simulink model "ATRIAS_vnmc"  (R2015a)
settings: Solver=ode45  StartTime=0.0  StopTime=60  FixedStep=1e-3  MinStep=1e-6  RelTol=1e-3  AbsTol=1e-4
values from neighbouring files (symbols this model uses):
  initial_boom_yaw = initial_boom_yaw + delta_yaw0    [run_model.m]
  max_floor_diff = cost_fun_opts.max_floor_diff    [opt_cmaes.m]    (also in run_model.m; set_all_params_simple.m = 0)
  noise_on_off = cost_fun_opts.noise_on_off    [opt_cmaes.m]    (also in run_model.m; set_all_params_simple.m = 0)
  noise_seed = cost_fun_opts.noise_seed    [opt_cmaes.m]    (also in run_model.m; set_all_params_simple.m = 1)
  noise_variance = cost_fun_opts.noise_variance    [opt_cmaes.m]    (also in run_model.m; set_all_params_simple.m = 0.000174532925199)
  SEA_swing_ctrl_on_off = cost_fun_opts.SEA_swing_ctrl_on_off    [opt_cmaes.m]    (also in run_model.m; set_all_params_simple.m = 0)
  sim_t = simout.twalk    [run_model.m]
  steady_dist = cost_fun_opts.steady_dist    [opt_cmaes.m]    (also in run_model.m; set_all_params_simple.m = 10)
  ts_anim = 0.0333    [run_model.m]
undefined symbols (not defined in the file or in its folder): A1_notch_f1, A2_notch_f1, A_lpf_dtau, A_lpf_velocity, B1_lpf_dtau, B1_lpf_velocity, B1_notch_f1, B2_lpf_dtau, B2_lpf_velocity, B2_notch_f1, b_hmotor, b_leg_spring, b_rotor, base_color_d, boom_color_d, boom_mount_to_center_diagonal, breakaway_friction, c, c_jointstop, com_height_offset, contactThr, coulomb_friction, CtrlPar_theta0, D12_S, D12_T, d_com, ddx_max, ddy_max, delta_phi_max, delta_phi_max_buffer, delta_phi_max_dropoff, delta_phi_min, des_forward_velocity, DS_width, dtau_des_max, dtheta0_vmc, dx0_vmc, dy_max, eref, fblink_color_d, fcut_acceleration, floor_color_d, floor_tile_width, floor_zero_height, FmaxBFSH, FmaxGLU, FmaxHAM, FmaxHFL, FmaxRF, FmaxVAS, FPCtrlPar, friction_linear_zone, g, gain_nodes_sea_torque, gamma_stance_thr, gamma_swing_thr, hip_height, HIP_MTR_MAX_CONT_TORQUE, HIP_MTR_MAX_TORQUE, hshaft_color_d ... (+236)
libraries: sm_lib x280, nesl_utility x174, simulink x114, simulink_extras x58, fl_lib x16, mblibv1 x2, dspswit3 x2
(part 9 of 23)

== system ATRIAS_vnmc/control/Virtual Model Control/Flight PD ==
  R Back Gear [rad rad/s] : Inport
  R Front Gear [rad rad/s] : Inport  Port=2
  L Back Gear [rad rad/s] : Inport  Port=3
  L Front Gear [rad rad/s] : Inport  Port=4
  R Length des [m] : Inport  Port=5
  R Gamma des [m] : Inport  Port=6
  L Length des [m] : Inport  Port=7
  L Angle des [m] : Inport  Port=8
  theta [rad] : Inport  Port=9
  Avoid Hitting Mechanical Limits1 : MATLAB Function  TreatAsAtomicUnit=on
  Avoid Hitting Mechanical Limits2 : MATLAB Function  TreatAsAtomicUnit=on
  Back/Front Motor PD1 : Subsystem
  Back/Front Motor PD2 : Subsystem
  Constant{3,5,7..12} (8 alike) : Constant  Value=0
  Demux{1..4} (4 alike) : Demux  Outputs=2
  Mux{1..9,11} (10 alike) : Mux  Inputs=2
  Sum : Sum  Inputs=|+-
  Sum1 : Sum  Inputs=-+|
  Virtual Leg to Four Bar1 : MATLAB Function  TreatAsAtomicUnit=on
  Virtual Leg to Four Bar2 : MATLAB Function  TreatAsAtomicUnit=on
  R cmd [Nm] [back front] : Outport
  L cmd [Nm] [back front] : Outport  Port=2
  wires:
  Virtual Leg to Four Bar1/1(back) -> Avoid Hitting Mechanical Limits1/1(back_desired)
  Virtual Leg to Four Bar1/2(dback) -> Avoid Hitting Mechanical Limits1/2(dback_desired)
  Virtual Leg to Four Bar1/3(ddback) -> Avoid Hitting Mechanical Limits1/3(ddback_desired)
  Virtual Leg to Four Bar1/4(front) -> Avoid Hitting Mechanical Limits1/4(front_desired)
  Virtual Leg to Four Bar1/5(dfront) -> Avoid Hitting Mechanical Limits1/5(dfront_desired)
  Virtual Leg to Four Bar1/6(ddfront) -> Avoid Hitting Mechanical Limits1/6(ddfront_desired)
  Mux5/1 -> Back/Front Motor PD1/1(Desired Position [rad] [back front])
  Avoid Hitting Mechanical Limits1/2(front_cmd) -> Mux5/2
  Avoid Hitting Mechanical Limits1/1(back_cmd) -> Mux5/1
  Avoid Hitting Mechanical Limits1/3(dback_cmd) -> Mux6/1
  Avoid Hitting Mechanical Limits1/4(dfront_cmd) -> Mux6/2
  Avoid Hitting Mechanical Limits1/5(ddback_cmd) -> Mux7/1
  Avoid Hitting Mechanical Limits1/6(ddfront_cmd) -> Mux7/2
  Mux6/1 -> Back/Front Motor PD1/2(Desired Velocity [rad/s] [back front])
  Mux7/1 -> Back/Front Motor PD1/3(Desired Acceleration [rad/s^2] [back front])
  R Length des [m]/1 -> Virtual Leg to Four Bar1/1(l_leg)
  Constant7/1 -> Virtual Leg to Four Bar1/2(dl_leg)
  Constant9/1 -> Virtual Leg to Four Bar1/5(dphi)
  Constant10/1 -> Virtual Leg to Four Bar1/6(ddphi)
  Constant8/1 -> Virtual Leg to Four Bar1/3(ddl_leg)
  Mux11/1 -> Back/Front Motor PD1/5(Measured Velocity [rad/s] [back front])
  Demux2/2 -> Mux11/2
  Mux4/1 -> Back/Front Motor PD1/4(Measured Position [rad] [back front])
  Demux3/2 -> Mux11/1
  Demux3/1 -> Mux4/1
  Demux2/1 -> Mux4/2
  R Front Gear [rad rad/s]/1 -> Demux2/1
  R Back Gear [rad rad/s]/1 -> Demux3/1
  Virtual Leg to Four Bar2/1(back) -> Avoid Hitting Mechanical Limits2/1(back_desired)
  Virtual Leg to Four Bar2/2(dback) -> Avoid Hitting Mechanical Limits2/2(dback_desired)
  Virtual Leg to Four Bar2/3(ddback) -> Avoid Hitting Mechanical Limits2/3(ddback_desired)
  Virtual Leg to Four Bar2/4(front) -> Avoid Hitting Mechanical Limits2/4(front_desired)
  Virtual Leg to Four Bar2/5(dfront) -> Avoid Hitting Mechanical Limits2/5(dfront_desired)
  Virtual Leg to Four Bar2/6(ddfront) -> Avoid Hitting Mechanical Limits2/6(ddfront_desired)
  Mux3/1 -> Back/Front Motor PD2/1(Desired Position [rad] [back front])
  Avoid Hitting Mechanical Limits2/2(front_cmd) -> Mux3/2
  Avoid Hitting Mechanical Limits2/1(back_cmd) -> Mux3/1
  Avoid Hitting Mechanical Limits2/3(dback_cmd) -> Mux8/1
  Avoid Hitting Mechanical Limits2/4(dfront_cmd) -> Mux8/2
  Avoid Hitting Mechanical Limits2/5(ddback_cmd) -> Mux9/1
  Avoid Hitting Mechanical Limits2/6(ddfront_cmd) -> Mux9/2
  Mux8/1 -> Back/Front Motor PD2/2(Desired Velocity [rad/s] [back front])
  Mux9/1 -> Back/Front Motor PD2/3(Desired Acceleration [rad/s^2] [back front])
  Constant5/1 -> Virtual Leg to Four Bar2/2(dl_leg)
  Constant12/1 -> Virtual Leg to Four Bar2/5(dphi)
  Constant3/1 -> Virtual Leg to Four Bar2/6(ddphi)
  Constant11/1 -> Virtual Leg to Four Bar2/3(ddl_leg)
  Mux1/1 -> Back/Front Motor PD2/5(Measured Velocity [rad/s] [back front])
  Demux1/2 -> Mux1/2
  Mux2/1 -> Back/Front Motor PD2/4(Measured Position [rad] [back front])
  Demux4/2 -> Mux1/1
  Demux4/1 -> Mux2/1
  Demux1/1 -> Mux2/2
  L Front Gear [rad rad/s]/1 -> Demux1/1
  L Back Gear [rad rad/s]/1 -> Demux4/1
  Back/Front Motor PD1/1(Commanded Torque [Nm] [back front]) -> R cmd [Nm] [back front]/1
  Back/Front Motor PD2/1(Commanded Torque [Nm] [back front]) -> L cmd [Nm] [back front]/1
  R Gamma des [m]/1 -> Sum/1
  L Length des [m]/1 -> Virtual Leg to Four Bar2/1(l_leg)
  L Angle des [m]/1 -> Sum1/2
  Sum/1 -> Virtual Leg to Four Bar1/4(phi)
  theta [rad]/1 -> Sum/2, Sum1/1
  Sum1/1 -> Virtual Leg to Four Bar2/4(phi)

== system ATRIAS_vnmc/control/Virtual Model Control/Swing Leg Behavior1 ==
  note: Leg Angle
  note: Leg Length
  note: Open-Loop Swing Trajectory
  note: Convert to
      | four-bar angles
  note: Position control the
      | individual four bar segments
  Swing Back Gear [rad rad/s] : Inport
  Swing Front Gear [rad rad/s] : Inport  Port=2
  Stance Leg Angle [rad] : Inport  Port=3
  Horizontal Single Support Distance [m] : Inport  Port=4
  Swing Leg Length [m] : Inport  Port=5
  Swing Leg Angle [rad] : Inport  Port=6
  COM Forward Velocity [m/s] : Inport  Port=7
  theta [rad rad/s] : Inport  Port=8
  Swing Leg Stance (VMC) [0/1] : Inport  Port=9
  Avoid Hitting Mechanical Limits : MATLAB Function  TreatAsAtomicUnit=on
  Back/Front Motor PD : Subsystem
  Clock : Clock
  Clock1 : Clock
  Constant1 : Constant  Value=nominal_swing_time
  Constant10 : Constant  Value=nominal_swing_time
  Constant11 : Constant  Value=max_gamma_velocity
  Constant12 : Constant  Value=max_gamma_acceleration
  Constant13 : Constant  Value=max_leg_velocity
  Constant14 : Constant  Value=max_leg_acceleration
  Constant2 : Constant  Commented=on  Value=gamma_swing_thr
  Constant6 : Constant  Value=leg_length_retract
  Constant7 : Constant  Value=leg_length_max+leg_ground_penetration
  Constant8 : Constant  Value=2*pi-gamma_swing_thr
  Constant9 : Constant  Commented=on  Value=eps
  Demux1 : Demux
  Demux2 : Demux  Outputs=2
  Demux3 : Demux  Outputs=2
  Demux4 : Demux
  Demux5 : Demux  Outputs=2
  Detect Change : simulink/Logic and Bit Operations/Detect Change  vinit=1  InputProcessing=Inherited  OutDataTypeStr=boolean
  Divide : Product  Commented=on  Inputs=*/
  Enter Swing or Stance : simulink/Logic and Bit Operations/Detect Change  vinit=1  InputProcessing=Inherited  OutDataTypeStr=boolean
  Hold Values : Subsystem
  Hold Values1 : Subsystem
  Leg Angle Trajectory : MATLAB Function  TreatAsAtomicUnit=on
  Leg Length Trajectory : MATLAB Function  TreatAsAtomicUnit=on
  Logical Operator : Logic  Operator=OR  AllPortsSameDT=off  OutDataTypeStr=boolean
  Mux : Mux
  Mux{1..4,11} (5 alike) : Mux  Inputs=2
  Mux5 : Mux
  Saturation : Saturate  Commented=on  UpperLimit=max_swing_time/2  LowerLimit=min_swing_time/2
  Saturation1 : Saturate  Commented=on  UpperLimit=2  LowerLimit=0.5
  Saturation2 : Saturate  Commented=on  UpperLimit=max_swing_time  LowerLimit=min_swing_time
  Sum{1..2,4..5} (4 alike) : Sum  Inputs=|+-
  Sum3 : Sum  Commented=on  Inputs=|++
  Sum6 : Sum  Inputs=|++
  Sum7 : Sum  Inputs=|++
  Switch : Switch  Criteria=u2 ~= 0
  Switch1 : Switch  Commented=on  Criteria=u2 ~= 0
  Terminator1 : Terminator  Commented=on
  Vertical/Trailing Swing Leg : simulink/Logic and Bit Operations/Compare To Constant  relop=<  const=pi  OutDataTypeStr=boolean
  Virtual Leg to Four Bar : MATLAB Function  TreatAsAtomicUnit=on
  half : Gain  Gain=1/2
  Secondary Back/Front Motor Torque [Nm Nm] : Outport
  Desired Leg Length [m] : Outport  Port=2
  Desired Leg Length Velocity [m/s] : Outport  Port=3
  Desired Leg Length Acceleration [m/s^2] : Outport  Port=4
  Desired Global Leg Angle [m] : Outport  Port=5
  Desired Global Leg Angle Velocity [m/s] : Outport  Port=6
  Desired Global Leg Angle Acceleration [m/s^2] : Outport  Port=7
  wires:
  Detect Change/1 -> Logical Operator/1
  Sum7/1 -> Desired Global Leg Angle Velocity [m/s]/1
  Sum6/1 -> Desired Global Leg Angle [m]/1
  Constant2/1 -> Switch1/1
  Constant1/1 -> Mux5/2
  [ddphi_swing] -> Desired Global Leg Angle Acceleration [m/s^2]/1
  [dphi_swing] -> Sum7/1
  [phi_swing] -> Sum6/1
  [ddl_leg_swing] -> Desired Leg Length Acceleration [m/s^2]/1
  [dl_leg_swing] -> Desired Leg Length Velocity [m/s]/1
  [l_leg_swing] -> Desired Leg Length [m]/1
  half/1 -> Mux/2
  Constant13/1 -> Leg Length Trajectory/5(max_leg_velocity)
  Constant14/1 -> Leg Length Trajectory/6(max_leg_acceleration)
  Constant12/1 -> Leg Angle Trajectory/6(max_gamma_acceleration)
  Constant11/1 -> Leg Angle Trajectory/5(max_gamma_velocity)
  Sum5/1 -> [dphi_swing]
  Demux5/2 -> Sum5/2, Sum7/2
  Demux5/1 -> Sum4/2, Sum6/2
  theta [rad rad/s]/1 -> Demux5/1
  Sum4/1 -> [phi_swing]
  Stance Leg Angle [rad]/1 -> Terminator1/1
  Constant10/1 -> half/1  "dt_sat"
  Saturation1/1 -> Sum3/1
  Constant9/1 -> Sum3/2
  Sum3/1 -> Divide/2
  Constant8/1 -> Mux5/3  "target leg angle"
  Swing Leg Angle [rad]/1 -> Vertical/Trailing Swing Leg/1, Mux5/4
  Clock1/1 -> Sum1/1, Mux5/1
  Sum1/1 -> Leg Angle Trajectory/1(t)
  Demux1/1 -> Sum1/2
  Demux1/2 -> Leg Angle Trajectory/4(t_trajectory)  "tmax"
  Demux1/3 -> Leg Angle Trajectory/3(gamma_final)
  Demux1/4 -> Leg Angle Trajectory/2(gamma_initial)
  Mux5/1 -> Hold Values1/1(in)
  Hold Values1/1(out) -> Demux1/1
  Leg Angle Trajectory/3(ddgamma) -> [ddphi_swing]  "ddgamma"
  Leg Angle Trajectory/2(dgamma) -> Sum5/1
  Leg Angle Trajectory/1(gamma) -> Sum4/1  "gamma"
  Logical Operator/1 -> Hold Values/Trigger
  Horizontal Single Support Distance [m]/1 -> Divide/1
  COM Forward Velocity [m/s]/1 -> Saturation1/1
  Switch/1 -> Mux/3
  Vertical/Trailing Swing Leg/1 -> Detect Change/1, Switch/2
  Constant7/1 -> Switch/1
  Constant6/1 -> Switch/3
  Enter Swing or Stance/1 -> Hold Values1/Trigger, Logical Operator/2
  Swing Leg Stance (VMC) [0/1]/1 -> Enter Swing or Stance/1, Switch1/2
  Swing Leg Length [m]/1 -> Mux/4
  Clock/1 -> Sum2/1, Mux/1
  Sum2/1 -> Leg Length Trajectory/1(t)
  Demux4/1 -> Sum2/2
  Demux4/2 -> Leg Length Trajectory/4(t_trajectory)
  Demux4/3 -> Leg Length Trajectory/3(l_leg_final)
  Demux4/4 -> Leg Length Trajectory/2(l_leg_initial)
  Mux/1 -> Hold Values/1(in)
  Hold Values/1(out) -> Demux4/1
  Leg Length Trajectory/3(ddl_leg) -> [ddl_leg_swing]
  Leg Length Trajectory/2(dl_leg) -> [dl_leg_swing]
  Leg Length Trajectory/1(l_leg) -> [l_leg_swing]
  [ddphi_swing] -> Virtual Leg to Four Bar/6(ddphi)
  [dphi_swing] -> Virtual Leg to Four Bar/5(dphi)
  [phi_swing] -> Virtual Leg to Four Bar/4(phi)
  [ddl_leg_swing] -> Virtual Leg to Four Bar/3(ddl_leg)
  [dl_leg_swing] -> Virtual Leg to Four Bar/2(dl_leg)
  [l_leg_swing] -> Virtual Leg to Four Bar/1(l_leg)
  Mux3/1 -> Back/Front Motor PD/3(Desired Acceleration [rad/s^2] [back front])
  Mux2/1 -> Back/Front Motor PD/2(Desired Velocity [rad/s] [back front])
  Avoid Hitting Mechanical Limits/6(ddfront_cmd) -> Mux3/2
  Avoid Hitting Mechanical Limits/5(ddback_cmd) -> Mux3/1
  Avoid Hitting Mechanical Limits/4(dfront_cmd) -> Mux2/2
  Avoid Hitting Mechanical Limits/3(dback_cmd) -> Mux2/1
  Swing Back Gear [rad rad/s]/1 -> Demux3/1
  Swing Front Gear [rad rad/s]/1 -> Demux2/1
  Demux2/1 -> Mux4/2
  Avoid Hitting Mechanical Limits/1(back_cmd) -> Mux1/1
  Avoid Hitting Mechanical Limits/2(front_cmd) -> Mux1/2
  Demux3/1 -> Mux4/1
  Demux3/2 -> Mux11/1
  Mux1/1 -> Back/Front Motor PD/1(Desired Position [rad] [back front])
  Mux4/1 -> Back/Front Motor PD/4(Measured Position [rad] [back front])
  Demux2/2 -> Mux11/2
  Mux11/1 -> Back/Front Motor PD/5(Measured Velocity [rad/s] [back front])
  Virtual Leg to Four Bar/6(ddfront) -> Avoid Hitting Mechanical Limits/6(ddfront_desired)
  Virtual Leg to Four Bar/5(dfront) -> Avoid Hitting Mechanical Limits/5(dfront_desired)
  Virtual Leg to Four Bar/4(front) -> Avoid Hitting Mechanical Limits/4(front_desired)
  Virtual Leg to Four Bar/3(ddback) -> Avoid Hitting Mechanical Limits/3(ddback_desired)
  Virtual Leg to Four Bar/2(dback) -> Avoid Hitting Mechanical Limits/2(dback_desired)
  Virtual Leg to Four Bar/1(back) -> Avoid Hitting Mechanical Limits/1(back_desired)
  Back/Front Motor PD/1(Commanded Torque [Nm] [back front]) -> Secondary Back/Front Motor Torque [Nm Nm]/1

== system ATRIAS_vnmc/control/Virtual Model Control/Swing Leg Behavior2 ==
  note: Position control the
      | individual four bar segments
  note: Convert to
      | four-bar angles
  note: Open-Loop Swing Trajectory
  note: Leg Length
  note: Leg Angle
  Swing Back Gear [rad rad/s] : Inport
  Swing Front Gear [rad rad/s] : Inport  Port=2
  Stance Leg Angle [rad] : Inport  Port=3
  Horizontal Single Support Distance [m] : Inport  Port=4
  Swing Leg Length [m] : Inport  Port=5
  Swing Leg Angle [rad] : Inport  Port=6
  COM Forward Velocity [m/s] : Inport  Port=7
  theta [rad rad/s] : Inport  Port=8
  Swing Leg Stance (VMC) [0/1] : Inport  Port=9
  Add : Sum  Inputs=+-
  Add1 : Sum
  Add2 : Sum  Inputs=+-
  Avoid Hitting Mechanical Limits : MATLAB Function  TreatAsAtomicUnit=on
  Back/Front Motor PD : Subsystem
  Clock : Clock
  Clock1 : Clock
  Constant1 : Constant  Value=nominal_swing_time
  Constant10 : Constant  Value=nominal_swing_time
  Constant11 : Constant  Value=max_gamma_velocity
  Constant12 : Constant  Value=max_gamma_acceleration
  Constant13 : Constant  Value=max_leg_velocity
  Constant14 : Constant  Value=max_leg_acceleration
  Constant2 : Constant  Value=2*pi
  Constant3 : Constant  Value=hip_height
  Constant5 : Constant  Value=leg_ground_penetration
  Constant6 : Constant  Value=leg_clearance
  Constant9 : Constant  Commented=on  Value=eps
  Demux1 : Demux
  Demux2 : Demux  Outputs=2
  Demux3 : Demux  Outputs=2
  Demux4 : Demux
  Demux5 : Demux  Outputs=2
  Detect Change : simulink/Logic and Bit Operations/Detect Change  vinit=1  InputProcessing=Inherited  OutDataTypeStr=boolean
  Divide : Product  Commented=on  Inputs=*/
  Enter Swing or Stance : simulink/Logic and Bit Operations/Detect Change  vinit=1  InputProcessing=Inherited  OutDataTypeStr=boolean
  Hold Values : Subsystem
  Hold Values1 : Subsystem
  Leg Angle Trajectory : MATLAB Function  TreatAsAtomicUnit=on
  Leg Length Trajectory : MATLAB Function  TreatAsAtomicUnit=on
  Logical Operator : Logic  Operator=OR  AllPortsSameDT=off  OutDataTypeStr=boolean
  Mux : Mux
  Mux{1..4,11} (5 alike) : Mux  Inputs=2
  Mux5 : Mux
  Saturation : Saturate  Commented=on  UpperLimit=max_swing_time/2  LowerLimit=min_swing_time/2
  Saturation1 : Saturate  Commented=on  UpperLimit=2  LowerLimit=0.5
  Saturation2 : Saturate  Commented=on  UpperLimit=max_swing_time  LowerLimit=min_swing_time
  Sum{1..2,4..5} (4 alike) : Sum  Inputs=|+-
  Sum3 : Sum  Commented=on  Inputs=|++
  Sum6 : Sum  Inputs=|++
  Sum7 : Sum  Inputs=|++
  Switch : Switch  Criteria=u2 ~= 0
  Terminator1 : Terminator
  Terminator2 : Terminator
  Terminator3 : Terminator
  Vertical/Trailing Swing Leg : simulink/Logic and Bit Operations/Compare To Constant  relop=<  const=pi  OutDataTypeStr=boolean
  Virtual Leg to Four Bar : MATLAB Function  TreatAsAtomicUnit=on
  half : Gain  Gain=1/2
  Secondary Back/Front Motor Torque [Nm Nm] : Outport
  Desired Leg Length [m] : Outport  Port=2
  Desired Leg Length Velocity [m/s] : Outport  Port=3
  Desired Leg Length Acceleration [m/s^2] : Outport  Port=4
  Desired Global Leg Angle [m] : Outport  Port=5
  Desired Global Leg Angle Velocity [m/s] : Outport  Port=6
  Desired Global Leg Angle Acceleration [m/s^2] : Outport  Port=7
  wires:
  Add2/1 -> Mux5/3
  Constant2/1 -> Add2/1
  [gamma_max] -> Add2/2
  [leg_length_max] -> Add1/1
  Constant5/1 -> Add1/2
  Constant3/1 -> Add/1
  Add/1 -> Switch/3
  Back/Front Motor PD/1(Commanded Torque [Nm] [back front]) -> Secondary Back/Front Motor Torque [Nm Nm]/1
  Virtual Leg to Four Bar/1(back) -> Avoid Hitting Mechanical Limits/1(back_desired)
  Virtual Leg to Four Bar/2(dback) -> Avoid Hitting Mechanical Limits/2(dback_desired)
  Virtual Leg to Four Bar/3(ddback) -> Avoid Hitting Mechanical Limits/3(ddback_desired)
  Virtual Leg to Four Bar/4(front) -> Avoid Hitting Mechanical Limits/4(front_desired)
  Virtual Leg to Four Bar/5(dfront) -> Avoid Hitting Mechanical Limits/5(dfront_desired)
  Virtual Leg to Four Bar/6(ddfront) -> Avoid Hitting Mechanical Limits/6(ddfront_desired)
  Mux11/1 -> Back/Front Motor PD/5(Measured Velocity [rad/s] [back front])
  Demux2/2 -> Mux11/2
  Mux4/1 -> Back/Front Motor PD/4(Measured Position [rad] [back front])
  Mux1/1 -> Back/Front Motor PD/1(Desired Position [rad] [back front])
  Demux3/2 -> Mux11/1
  Demux3/1 -> Mux4/1
  Avoid Hitting Mechanical Limits/2(front_cmd) -> Mux1/2
  Avoid Hitting Mechanical Limits/1(back_cmd) -> Mux1/1
  Demux2/1 -> Mux4/2
  Swing Front Gear [rad rad/s]/1 -> Demux2/1
  Swing Back Gear [rad rad/s]/1 -> Demux3/1
  Avoid Hitting Mechanical Limits/3(dback_cmd) -> Mux2/1
  Avoid Hitting Mechanical Limits/4(dfront_cmd) -> Mux2/2
  Avoid Hitting Mechanical Limits/5(ddback_cmd) -> Mux3/1
  Avoid Hitting Mechanical Limits/6(ddfront_cmd) -> Mux3/2
  Mux2/1 -> Back/Front Motor PD/2(Desired Velocity [rad/s] [back front])
  Mux3/1 -> Back/Front Motor PD/3(Desired Acceleration [rad/s^2] [back front])
  [l_leg_swing] -> Virtual Leg to Four Bar/1(l_leg)
  [dl_leg_swing] -> Virtual Leg to Four Bar/2(dl_leg)
  [ddl_leg_swing] -> Virtual Leg to Four Bar/3(ddl_leg)
  [phi_swing] -> Virtual Leg to Four Bar/4(phi)
  [dphi_swing] -> Virtual Leg to Four Bar/5(dphi)
  [ddphi_swing] -> Virtual Leg to Four Bar/6(ddphi)
  Leg Length Trajectory/1(l_leg) -> [l_leg_swing]
  Leg Length Trajectory/2(dl_leg) -> [dl_leg_swing]
  Leg Length Trajectory/3(ddl_leg) -> [ddl_leg_swing]
  Hold Values/1(out) -> Demux4/1
  Mux/1 -> Hold Values/1(in)
  Demux4/4 -> Leg Length Trajectory/2(l_leg_initial)
  Demux4/3 -> Leg Length Trajectory/3(l_leg_final)
  Demux4/2 -> Leg Length Trajectory/4(t_trajectory)
  Demux4/1 -> Sum2/2
  Sum2/1 -> Leg Length Trajectory/1(t)
  Clock/1 -> Mux/1, Sum2/1
  Swing Leg Length [m]/1 -> Mux/4
  Swing Leg Stance (VMC) [0/1]/1 -> Enter Swing or Stance/1
  Enter Swing or Stance/1 -> Logical Operator/2, Hold Values1/Trigger
  Constant6/1 -> Add/2
  Add1/1 -> Switch/1
  Vertical/Trailing Swing Leg/1 -> Switch/2, Detect Change/1
  Switch/1 -> Mux/3
  COM Forward Velocity [m/s]/1 -> Terminator3/1
  Horizontal Single Support Distance [m]/1 -> Terminator2/1
  Logical Operator/1 -> Hold Values/Trigger
  Leg Angle Trajectory/1(gamma) -> Sum4/1  "gamma"
  Leg Angle Trajectory/2(dgamma) -> Sum5/1
  Leg Angle Trajectory/3(ddgamma) -> [ddphi_swing]  "ddgamma"
  Hold Values1/1(out) -> Demux1/1
  Mux5/1 -> Hold Values1/1(in)
  Demux1/4 -> Leg Angle Trajectory/2(gamma_initial)
  Demux1/3 -> Leg Angle Trajectory/3(gamma_final)
  Demux1/2 -> Leg Angle Trajectory/4(t_trajectory)  "tmax"
  Demux1/1 -> Sum1/2
  Sum1/1 -> Leg Angle Trajectory/1(t)
  Clock1/1 -> Sum1/1, Mux5/1
  Swing Leg Angle [rad]/1 -> Mux5/4, Vertical/Trailing Swing Leg/1
  Sum3/1 -> Divide/2
  Constant9/1 -> Sum3/2
  Saturation1/1 -> Sum3/1
  Constant10/1 -> half/1  "dt_sat"
  Stance Leg Angle [rad]/1 -> Terminator1/1
  Sum4/1 -> [phi_swing]
  theta [rad rad/s]/1 -> Demux5/1
  Demux5/1 -> Sum6/2, Sum4/2
  Demux5/2 -> Sum7/2, Sum5/2
  Sum5/1 -> [dphi_swing]
  Constant11/1 -> Leg Angle Trajectory/5(max_gamma_velocity)
  Constant12/1 -> Leg Angle Trajectory/6(max_gamma_acceleration)
  Constant14/1 -> Leg Length Trajectory/6(max_leg_acceleration)
  Constant13/1 -> Leg Length Trajectory/5(max_leg_velocity)
  half/1 -> Mux/2
  [l_leg_swing] -> Desired Leg Length [m]/1
  [dl_leg_swing] -> Desired Leg Length Velocity [m/s]/1
  [ddl_leg_swing] -> Desired Leg Length Acceleration [m/s^2]/1
  [phi_swing] -> Sum6/1
  [dphi_swing] -> Sum7/1
  [ddphi_swing] -> Desired Global Leg Angle Acceleration [m/s^2]/1
  Constant1/1 -> Mux5/2
  Sum6/1 -> Desired Global Leg Angle [m]/1
  Sum7/1 -> Desired Global Leg Angle Velocity [m/s]/1
  Detect Change/1 -> Logical Operator/1

== system ATRIAS_vnmc/control/Virtual Model Control/Swing Leg Behavior3 ==
  note: Leg Angle
  note: Leg Length
  note: Open-Loop Swing Trajectory
  note: Convert to
      | four-bar angles
  note: Position control the
      | individual four bar segments
  Swing Back Gear [rad rad/s] : Inport
  Swing Front Gear [rad rad/s] : Inport  Port=2
  Stance Leg Angle [rad] : Inport  Port=3
  Horizontal Single Support Distance [m] : Inport  Port=4
  Swing Leg Length [m] : Inport  Port=5
  Swing Leg Angle [rad] : Inport  Port=6
  COM Forward Velocity [m/s] : Inport  Port=7
  theta [rad rad/s] : Inport  Port=8
  Swing Leg Stance (VMC) [0/1] : Inport  Port=9
  Add : Sum  Inputs=+-
  Add1 : Sum  Inputs=+-
  Add2 : Sum  Inputs=+-
  Avoid Hitting Mechanical Limits : MATLAB Function  TreatAsAtomicUnit=on
  Back/Front Motor PD : Subsystem
  Clock : Clock
  Clock1 : Clock
  Constant1 : Constant  Value=nominal_swing_time
  Constant10 : Constant  Value=nominal_swing_time
  Constant11 : Constant  Value=max_gamma_velocity
  Constant12 : Constant  Value=max_gamma_acceleration
  Constant13 : Constant  Value=max_leg_velocity
  Constant14 : Constant  Value=max_leg_acceleration
  Constant2 : Constant  Value=2*pi
  Constant3 : Constant  Value=hip_height
  Constant5 : Constant  Value=leg_ground_penetration
  Constant6 : Constant  Value=leg_clearance
  Constant9 : Constant  Commented=on  Value=eps
  Demux1 : Demux
  Demux2 : Demux  Outputs=2
  Demux3 : Demux  Outputs=2
  Demux4 : Demux
  Demux5 : Demux  Outputs=2
  Detect Change : simulink/Logic and Bit Operations/Detect Change  vinit=1  InputProcessing=Inherited  OutDataTypeStr=boolean
  Divide : Product  Commented=on  Inputs=*/
  Enter Swing or Stance : simulink/Logic and Bit Operations/Detect Change  vinit=1  InputProcessing=Inherited  OutDataTypeStr=boolean
  Hold Values : Subsystem
  Hold Values1 : Subsystem
  Leg Angle Trajectory : MATLAB Function  TreatAsAtomicUnit=on
  Leg Length Trajectory : MATLAB Function  TreatAsAtomicUnit=on
  Logical Operator : Logic  Operator=OR  AllPortsSameDT=off  OutDataTypeStr=boolean
  Mux : Mux
  Mux{1..4,11} (5 alike) : Mux  Inputs=2
  Mux5 : Mux
  Saturation : Saturate  Commented=on  UpperLimit=max_swing_time/2  LowerLimit=min_swing_time/2
  Saturation1 : Saturate  Commented=on  UpperLimit=2  LowerLimit=0.5
  Saturation2 : Saturate  Commented=on  UpperLimit=max_swing_time  LowerLimit=min_swing_time
  Sum{1..2,4..5} (4 alike) : Sum  Inputs=|+-
  Sum3 : Sum  Commented=on  Inputs=|++
  Sum6 : Sum  Inputs=|++
  Sum7 : Sum  Inputs=|++
  Switch : Switch  Criteria=u2 ~= 0
  Terminator1 : Terminator
  Terminator2 : Terminator
  Terminator3 : Terminator
  Vertical/Trailing Swing Leg : simulink/Logic and Bit Operations/Compare To Constant  relop=<  const=pi  OutDataTypeStr=boolean
  Virtual Leg to Four Bar : MATLAB Function  TreatAsAtomicUnit=on
  half : Gain  Gain=1/2
  Secondary Back/Front Motor Torque [Nm Nm] : Outport
  Desired Leg Length [m] : Outport  Port=2
  Desired Leg Length Velocity [m/s] : Outport  Port=3
  Desired Leg Length Acceleration [m/s^2] : Outport  Port=4
  Desired Global Leg Angle [m] : Outport  Port=5
  Desired Global Leg Angle Velocity [m/s] : Outport  Port=6
  Desired Global Leg Angle Acceleration [m/s^2] : Outport  Port=7
  wires:
  Detect Change/1 -> Logical Operator/1
  Sum7/1 -> Desired Global Leg Angle Velocity [m/s]/1
  Sum6/1 -> Desired Global Leg Angle [m]/1
  Constant1/1 -> Mux5/2
  [ddphi_swing] -> Desired Global Leg Angle Acceleration [m/s^2]/1
  [dphi_swing] -> Sum7/1
  [phi_swing] -> Sum6/1
  [ddl_leg_swing] -> Desired Leg Length Acceleration [m/s^2]/1
  [dl_leg_swing] -> Desired Leg Length Velocity [m/s]/1
  [l_leg_swing] -> Desired Leg Length [m]/1
  half/1 -> Mux/2
  Constant13/1 -> Leg Length Trajectory/5(max_leg_velocity)
  Constant14/1 -> Leg Length Trajectory/6(max_leg_acceleration)
  Constant12/1 -> Leg Angle Trajectory/6(max_gamma_acceleration)
  Constant11/1 -> Leg Angle Trajectory/5(max_gamma_velocity)
  Sum5/1 -> [dphi_swing]
  Demux5/2 -> Sum5/2, Sum7/2
  Demux5/1 -> Sum4/2, Sum6/2
  theta [rad rad/s]/1 -> Demux5/1
  Sum4/1 -> [phi_swing]
  Stance Leg Angle [rad]/1 -> Terminator1/1
  Constant10/1 -> half/1  "dt_sat"
  Saturation1/1 -> Sum3/1
  Constant9/1 -> Sum3/2
  Sum3/1 -> Divide/2
  Swing Leg Angle [rad]/1 -> Vertical/Trailing Swing Leg/1, Mux5/4
  Clock1/1 -> Mux5/1, Sum1/1
  Sum1/1 -> Leg Angle Trajectory/1(t)
  Demux1/1 -> Sum1/2
  Demux1/2 -> Leg Angle Trajectory/4(t_trajectory)  "tmax"
  Demux1/3 -> Leg Angle Trajectory/3(gamma_final)
  Demux1/4 -> Leg Angle Trajectory/2(gamma_initial)
  Mux5/1 -> Hold Values1/1(in)
  Hold Values1/1(out) -> Demux1/1
  Leg Angle Trajectory/3(ddgamma) -> [ddphi_swing]  "ddgamma"
  Leg Angle Trajectory/2(dgamma) -> Sum5/1
  Leg Angle Trajectory/1(gamma) -> Sum4/1  "gamma"
  Logical Operator/1 -> Hold Values/Trigger
  Horizontal Single Support Distance [m]/1 -> Terminator2/1
  COM Forward Velocity [m/s]/1 -> Terminator3/1
  Switch/1 -> Mux/3
  Vertical/Trailing Swing Leg/1 -> Detect Change/1, Switch/2
  Add1/1 -> Switch/1
  Constant6/1 -> Add/2
  Enter Swing or Stance/1 -> Hold Values1/Trigger, Logical Operator/2
  Swing Leg Stance (VMC) [0/1]/1 -> Enter Swing or Stance/1
  Swing Leg Length [m]/1 -> Mux/4
  Clock/1 -> Sum2/1, Mux/1
  Sum2/1 -> Leg Length Trajectory/1(t)
  Demux4/1 -> Sum2/2
  Demux4/2 -> Leg Length Trajectory/4(t_trajectory)
  Demux4/3 -> Leg Length Trajectory/3(l_leg_final)
  Demux4/4 -> Leg Length Trajectory/2(l_leg_initial)
  Mux/1 -> Hold Values/1(in)
  Hold Values/1(out) -> Demux4/1
  Leg Length Trajectory/3(ddl_leg) -> [ddl_leg_swing]
  Leg Length Trajectory/2(dl_leg) -> [dl_leg_swing]
  Leg Length Trajectory/1(l_leg) -> [l_leg_swing]
  [ddphi_swing] -> Virtual Leg to Four Bar/6(ddphi)
  [dphi_swing] -> Virtual Leg to Four Bar/5(dphi)
  [phi_swing] -> Virtual Leg to Four Bar/4(phi)
  [ddl_leg_swing] -> Virtual Leg to Four Bar/3(ddl_leg)
  [dl_leg_swing] -> Virtual Leg to Four Bar/2(dl_leg)
  [l_leg_swing] -> Virtual Leg to Four Bar/1(l_leg)
  Mux3/1 -> Back/Front Motor PD/3(Desired Acceleration [rad/s^2] [back front])
  Mux2/1 -> Back/Front Motor PD/2(Desired Velocity [rad/s] [back front])
  Avoid Hitting Mechanical Limits/6(ddfront_cmd) -> Mux3/2
  Avoid Hitting Mechanical Limits/5(ddback_cmd) -> Mux3/1
  Avoid Hitting Mechanical Limits/4(dfront_cmd) -> Mux2/2
  Avoid Hitting Mechanical Limits/3(dback_cmd) -> Mux2/1
  Swing Back Gear [rad rad/s]/1 -> Demux3/1
  Swing Front Gear [rad rad/s]/1 -> Demux2/1
  Demux2/1 -> Mux4/2
  Avoid Hitting Mechanical Limits/1(back_cmd) -> Mux1/1
  Avoid Hitting Mechanical Limits/2(front_cmd) -> Mux1/2
  Demux3/1 -> Mux4/1
  Demux3/2 -> Mux11/1
  Mux1/1 -> Back/Front Motor PD/1(Desired Position [rad] [back front])
  Mux4/1 -> Back/Front Motor PD/4(Measured Position [rad] [back front])
  Demux2/2 -> Mux11/2
  Mux11/1 -> Back/Front Motor PD/5(Measured Velocity [rad/s] [back front])
  Virtual Leg to Four Bar/6(ddfront) -> Avoid Hitting Mechanical Limits/6(ddfront_desired)
  Virtual Leg to Four Bar/5(dfront) -> Avoid Hitting Mechanical Limits/5(dfront_desired)
  Virtual Leg to Four Bar/4(front) -> Avoid Hitting Mechanical Limits/4(front_desired)
  Virtual Leg to Four Bar/3(ddback) -> Avoid Hitting Mechanical Limits/3(ddback_desired)
  Virtual Leg to Four Bar/2(dback) -> Avoid Hitting Mechanical Limits/2(dback_desired)
  Virtual Leg to Four Bar/1(back) -> Avoid Hitting Mechanical Limits/1(back_desired)
  Back/Front Motor PD/1(Commanded Torque [Nm] [back front]) -> Secondary Back/Front Motor Torque [Nm Nm]/1
  Add/1 -> Switch/3
  Constant3/1 -> Add/1
  Constant5/1 -> Add1/2
  [leg_length_max] -> Add1/1
  [gamma_max] -> Add2/2
  Constant2/1 -> Add2/1
  Add2/1 -> Mux5/3

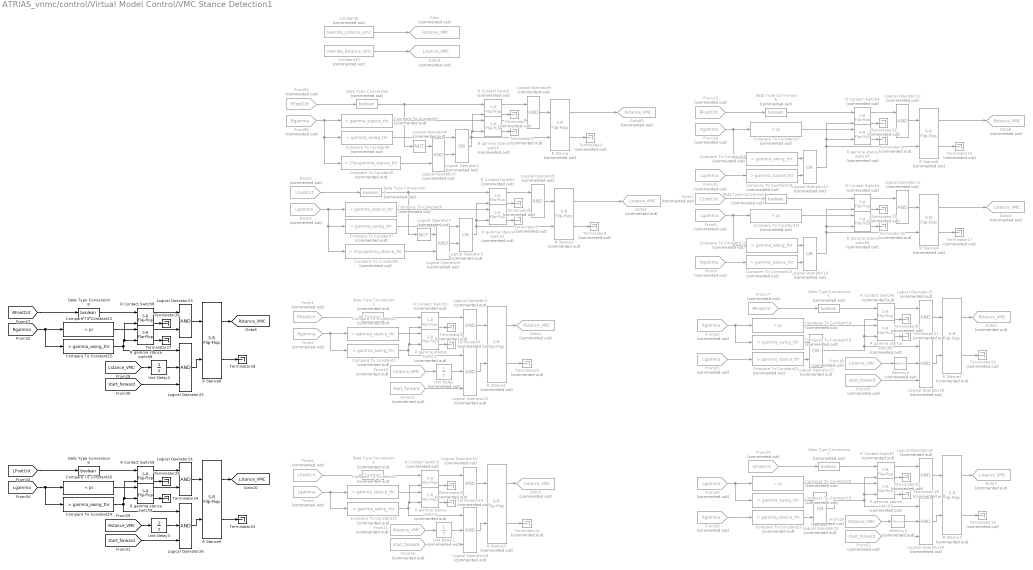
== system ATRIAS_vnmc/control/Virtual Model Control/VMC Stance Detection1 ==
  Compare To Constant{1,3,6,9} (4 alike) : simulink/Logic and Bit Operations/Compare To Constant  Commented=on  relop=<  const=gamma_stance_thr  OutDataTypeStr=boolean
  Compare To Constant{2,4,7,10,12,15..16,18} (8 alike) : simulink/Logic and Bit Operations/Compare To Constant  Commented=on  relop=>  const=gamma_swing_thr  OutDataTypeStr=boolean
  Compare To Constant{11,14,17,20} (4 alike) : simulink/Logic and Bit Operations/Compare To Constant  Commented=on  relop=<  const=pi  OutDataTypeStr=boolean
  Compare To Constant{13,19,21..22} (4 alike) : simulink/Logic and Bit Operations/Compare To Constant  Commented=on  relop=>  const=gamma_stance_thr  OutDataTypeStr=boolean
  Compare To Constant23 : simulink/Logic and Bit Operations/Compare To Constant  relop=<  const=pi  OutDataTypeStr=boolean
  Compare To Constant24 : simulink/Logic and Bit Operations/Compare To Constant  relop=>  const=gamma_swing_thr  OutDataTypeStr=boolean
  Compare To Constant25 : simulink/Logic and Bit Operations/Compare To Constant  relop=>  const=gamma_swing_thr  OutDataTypeStr=boolean
  Compare To Constant26 : simulink/Logic and Bit Operations/Compare To Constant  relop=<  const=pi  OutDataTypeStr=boolean
  Compare To Constant5 : simulink/Logic and Bit Operations/Compare To Constant  Commented=on  relop=>  const=2*pi-gamma_stance_thr  OutDataTypeStr=boolean
  Compare To Constant8 : simulink/Logic and Bit Operations/Compare To Constant  Commented=on  relop=>  const=2*pi-gamma_stance_thr  OutDataTypeStr=boolean
  Constant10 : Constant  Commented=on  Value=override_Rstance_vmc
  Constant9 : Constant  Commented=on  Value=override_Lstance_vmc
  Data Type Conversion{,1..7} (8 alike) : DataTypeConversion  Commented=on  OutDataTypeStr=boolean
  Data Type Conversion8 : DataTypeConversion  OutDataTypeStr=boolean
  Data Type Conversion9 : DataTypeConversion  OutDataTypeStr=boolean
  From{1,13,17,94} (4 alike) : From  Commented=on  GotoTag=RFootCnt  TagVisibility=global
  From10 : From  Commented=on  GotoTag=Lstance_VMC  TagVisibility=global
  From11 : From  Commented=on  GotoTag=Rstance_VMC  TagVisibility=global
  From{12,16,20..21} (4 alike) : From  Commented=on  GotoTag=start_forward  TagVisibility=global
  From{2,9,14,22,26,96} (6 alike) : From  Commented=on  GotoTag=Rgamma  TagVisibility=global
  From{4,6,8,15,24..25} (6 alike) : From  Commented=on  GotoTag=Lgamma  TagVisibility=global
  From18 : From  Commented=on  GotoTag=Lstance_VMC  TagVisibility=global
  From19 : From  Commented=on  GotoTag=Rstance_VMC  TagVisibility=global
  From{3,5,7,23} (4 alike) : From  Commented=on  GotoTag=LFootCnt  TagVisibility=global
  Goto{,1,5..6,60} (5 alike) : Goto  Commented=on  GotoTag=Rstance_VMC  TagVisibility=global
  Goto{2..4,7,9} (5 alike) : Goto  Commented=on  GotoTag=Lstance_VMC  TagVisibility=global
  Logical Operator{1,3,6,8..12,17..18} (10 alike) : Logic  Commented=on  AllPortsSameDT=off  OutDataTypeStr=boolean
  Logical Operator{2,5,13..14,21..22} (6 alike) : Logic  Commented=on  Operator=OR  AllPortsSameDT=off  OutDataTypeStr=boolean
  Logical Operator{15..16,19..20} (4 alike) : Logic  Commented=on  Inputs=3  AllPortsSameDT=off  OutDataTypeStr=boolean
  Logical Operator23 : Logic  AllPortsSameDT=off  OutDataTypeStr=boolean
  Logical Operator24 : Logic  AllPortsSameDT=off  OutDataTypeStr=boolean
  Logical Operator25 : Logic  Inputs=3  AllPortsSameDT=off  OutDataTypeStr=boolean
  Logical Operator26 : Logic  Inputs=3  AllPortsSameDT=off  OutDataTypeStr=boolean
  Logical Operator4 : Logic  Commented=on  Operator=NOT  AllPortsSameDT=off  OutDataTypeStr=boolean
  Logical Operator7 : Logic  Commented=on  Operator=NOT  AllPortsSameDT=off  OutDataTypeStr=boolean
  Memory2 : Memory  Commented=on
  Memory3 : Memory  Commented=on
  R Contact Switch{,1..7} (8 alike) : simulink_extras/Flip Flops/S-R Flip-Flop  Commented=on  initial_condition=0
  R Contact Switch8 : simulink_extras/Flip Flops/S-R Flip-Flop  initial_condition=0
  R Contact Switch9 : simulink_extras/Flip Flops/S-R Flip-Flop  initial_condition=0
  R Stance{,1..7} (8 alike) : simulink_extras/Flip Flops/S-R Flip-Flop  Commented=on  initial_condition=1
  R Stance8 : simulink_extras/Flip Flops/S-R Flip-Flop  initial_condition=1
  R Stance9 : simulink_extras/Flip Flops/S-R Flip-Flop  initial_condition=1
  R gamma stance switch{,1..7} (8 alike) : simulink_extras/Flip Flops/S-R Flip-Flop  Commented=on  initial_condition=0
  R gamma stance switch8 : simulink_extras/Flip Flops/S-R Flip-Flop  initial_condition=0
  R gamma stance switch9 : simulink_extras/Flip Flops/S-R Flip-Flop  initial_condition=0
  Terminator{,1..23} (24 alike) : Terminator  Commented=on
  Terminator{24..29} (6 alike) : Terminator
  Unit Delay : UnitDelay  Commented=on  InitialCondition=1  SampleTime=-1
  Unit Delay1 : UnitDelay  Commented=on  InitialCondition=1  SampleTime=-1
  Unit Delay2 : UnitDelay  InitialCondition=1  SampleTime=-1
  Unit Delay3 : UnitDelay  InitialCondition=1  SampleTime=-1
  tag scope: Lstance_VMC=global, Rstance_VMC=global
  wires:
  Compare To Constant22/1 -> Logical Operator22/2
  From26/1 -> Compare To Constant22/1
  Compare To Constant15/1 -> Logical Operator22/1
  Compare To Constant21/1 -> Logical Operator21/2
  Compare To Constant16/1 -> Logical Operator21/1
  From25/1 -> Compare To Constant21/1
  From21/1 -> Logical Operator20/3
  From20/1 -> Logical Operator19/3
  Memory3/1 -> Logical Operator20/2
  Memory2/1 -> Logical Operator19/2
  Logical Operator20/1 -> R Stance7/2
  From19/1 -> Memory3/1
  From18/1 -> Memory2/1
  Logical Operator19/1 -> R Stance5/2
  Data Type Conversion7/1 -> R Contact Switch7/1
  R gamma stance switch7/2 -> Terminator18/1
  R Contact Switch7/2 -> Terminator23/1
  R gamma stance switch7/1 -> Logical Operator18/2
  R Contact Switch7/1 -> Logical Operator18/1
  Logical Operator18/1 -> R Stance7/1
  From23/1 -> Data Type Conversion7/1
  R Stance7/2 -> Terminator19/1
  From24/1 -> Compare To Constant20/1, Compare To Constant15/1
  Logical Operator22/1 -> R gamma stance switch7/2, R Contact Switch7/2, Logical Operator20/1
  Compare To Constant20/1 -> R gamma stance switch7/1
  R Stance7/1 -> Goto7/1
  Data Type Conversion5/1 -> R Contact Switch6/1
  R gamma stance switch6/2 -> Terminator21/1
  R Contact Switch6/2 -> Terminator20/1
  R gamma stance switch6/1 -> Logical Operator17/2
  R Contact Switch6/1 -> Logical Operator17/1
  Logical Operator17/1 -> R Stance5/1
  From17/1 -> Data Type Conversion5/1
  R Stance5/2 -> Terminator22/1
  From22/1 -> Compare To Constant14/1, Compare To Constant16/1
  Logical Operator21/1 -> Logical Operator19/1, R gamma stance switch6/2, R Contact Switch6/2
  Compare To Constant14/1 -> R gamma stance switch6/1
  R Stance5/1 -> Goto5/1
  From16/1 -> Logical Operator16/3
  From12/1 -> Logical Operator15/3
  Unit Delay1/1 -> Logical Operator16/2
  Unit Delay/1 -> Logical Operator15/2
  Logical Operator16/1 -> R Stance3/2
  From11/1 -> Unit Delay1/1
  From10/1 -> Unit Delay/1
  Logical Operator15/1 -> R Stance1/2
  Compare To Constant12/1 -> Logical Operator14/1
  Compare To Constant13/1 -> Logical Operator14/2
  From9/1 -> Compare To Constant13/1
  Data Type Conversion4/1 -> R Contact Switch5/1
  R gamma stance switch5/2 -> Terminator16/1
  R Contact Switch5/2 -> Terminator13/1
  R gamma stance switch5/1 -> Logical Operator11/2
  R Contact Switch5/1 -> Logical Operator11/1
  Logical Operator11/1 -> R Stance4/1
  From7/1 -> Data Type Conversion4/1
  R Stance4/2 -> Terminator17/1
  From8/1 -> Compare To Constant11/1, Compare To Constant12/1
  Logical Operator14/1 -> R gamma stance switch5/2, R Contact Switch5/2, R Stance4/2
  Compare To Constant11/1 -> R gamma stance switch5/1
  R Stance4/1 -> Goto4/1
  Compare To Constant18/1 -> Logical Operator13/1
  Compare To Constant19/1 -> Logical Operator13/2
  From15/1 -> Compare To Constant19/1
  Data Type Conversion6/1 -> R Contact Switch4/1
  R gamma stance switch4/2 -> Terminator14/1
  R Contact Switch4/2 -> Terminator12/1
  R gamma stance switch4/1 -> Logical Operator12/2
  R Contact Switch4/1 -> Logical Operator12/1
  Logical Operator12/1 -> R Stance6/1
  From13/1 -> Data Type Conversion6/1
  R Stance6/2 -> Terminator15/1
  From14/1 -> Compare To Constant17/1, Compare To Constant18/1
  Logical Operator13/1 -> R gamma stance switch4/2, R Contact Switch4/2, R Stance6/2
  Compare To Constant17/1 -> R gamma stance switch4/1
  R Stance6/1 -> Goto6/1
  Data Type Conversion3/1 -> R Contact Switch3/1
  R gamma stance switch3/2 -> Terminator10/1
  R Contact Switch3/2 -> Terminator9/1
  R gamma stance switch3/1 -> Logical Operator10/2
  R Contact Switch3/1 -> Logical Operator10/1
  Logical Operator10/1 -> R Stance3/1
  From5/1 -> Data Type Conversion3/1
  R Stance3/2 -> Terminator11/1
  From6/1 -> Compare To Constant9/1, Compare To Constant10/1
  Compare To Constant10/1 -> R gamma stance switch3/2, R Contact Switch3/2, Logical Operator16/1
  Compare To Constant9/1 -> R gamma stance switch3/1
  R Stance3/1 -> Goto3/1
  Compare To Constant8/1 -> Logical Operator6/2
  Logical Operator7/1 -> Logical Operator6/1
  Logical Operator6/1 -> Logical Operator5/2
  Compare To Constant7/1 -> Logical Operator5/1
  Data Type Conversion2/1 -> R Contact Switch2/1, Logical Operator7/1
  R gamma stance switch2/2 -> Terminator7/1
  R Contact Switch2/2 -> Terminator6/1
  R gamma stance switch2/1 -> Logical Operator8/2
  R Contact Switch2/1 -> Logical Operator8/1
  Logical Operator8/1 -> R Stance2/1
  From3/1 -> Data Type Conversion2/1
  R Stance2/2 -> Terminator8/1
  From4/1 -> Compare To Constant6/1, Compare To Constant7/1, Compare To Constant8/1
  Logical Operator5/1 -> R Stance2/2, R gamma stance switch2/2, R Contact Switch2/2
  Compare To Constant6/1 -> R gamma stance switch2/1
  R Stance2/1 -> Goto2/1
  Compare To Constant5/1 -> Logical Operator3/2
  Logical Operator4/1 -> Logical Operator3/1
  Logical Operator3/1 -> Logical Operator2/2
  Compare To Constant4/1 -> Logical Operator2/1
  Data Type Conversion1/1 -> R Contact Switch1/1
  Data Type Conversion/1 -> R Contact Switch/1, Logical Operator4/1
  R gamma stance switch1/2 -> Terminator4/1
  R Contact Switch1/2 -> Terminator2/1
  R gamma stance switch1/1 -> Logical Operator1/2
  R Contact Switch1/1 -> Logical Operator1/1
  Logical Operator1/1 -> R Stance1/1
  From1/1 -> Data Type Conversion1/1
  R Stance1/2 -> Terminator5/1
  From2/1 -> Compare To Constant1/1, Compare To Constant2/1
  Compare To Constant2/1 -> R gamma stance switch1/2, R Contact Switch1/2, Logical Operator15/1
  Compare To Constant1/1 -> R gamma stance switch1/1
  R Stance1/1 -> Goto1/1
  R gamma stance switch/2 -> Terminator1/1
  R Contact Switch/2 -> Terminator/1
  R gamma stance switch/1 -> Logical Operator9/2
  R Contact Switch/1 -> Logical Operator9/1
  Logical Operator9/1 -> R Stance/1
  From94/1 -> Data Type Conversion/1
  R Stance/2 -> Terminator3/1
  From96/1 -> Compare To Constant3/1, Compare To Constant4/1, Compare To Constant5/1
  Logical Operator2/1 -> R Stance/2, R gamma stance switch/2, R Contact Switch/2
  Compare To Constant3/1 -> R gamma stance switch/1
  R Stance/1 -> Goto60/1
  Constant10/1 -> Goto9/1
  Constant9/1 -> Goto/1
  [start_forward] -> Logical Operator26/3
  [start_forward] -> Logical Operator25/3
  Unit Delay3/1 -> Logical Operator26/2
  Unit Delay2/1 -> Logical Operator25/2
  Logical Operator26/1 -> R Stance9/2
  [Rstance_VMC] -> Unit Delay3/1
  [Lstance_VMC] -> Unit Delay2/1
  Logical Operator25/1 -> R Stance8/2
  Data Type Conversion9/1 -> R Contact Switch9/1
  R gamma stance switch9/2 -> Terminator24/1
  R Contact Switch9/2 -> Terminator29/1
  R gamma stance switch9/1 -> Logical Operator24/2
  R Contact Switch9/1 -> Logical Operator24/1
  Logical Operator24/1 -> R Stance9/1
  [LFootCnt] -> Data Type Conversion9/1
  R Stance9/2 -> Terminator25/1
  [Lgamma] -> Compare To Constant26/1, Compare To Constant24/1
  Compare To Constant24/1 -> R gamma stance switch9/2, R Contact Switch9/2, Logical Operator26/1
  Compare To Constant26/1 -> R gamma stance switch9/1
  R Stance9/1 -> [Lstance_VMC]
  Data Type Conversion8/1 -> R Contact Switch8/1
  R gamma stance switch8/2 -> Terminator27/1
  R Contact Switch8/2 -> Terminator26/1
  R gamma stance switch8/1 -> Logical Operator23/2
  R Contact Switch8/1 -> Logical Operator23/1
  Logical Operator23/1 -> R Stance8/1
  [RFootCnt] -> Data Type Conversion8/1
  R Stance8/2 -> Terminator28/1
  [Rgamma] -> Compare To Constant23/1, Compare To Constant25/1
  Compare To Constant25/1 -> R gamma stance switch8/2, R Contact Switch8/2, Logical Operator25/1
  Compare To Constant23/1 -> R gamma stance switch8/1
  R Stance8/1 -> [Rstance_VMC]

== system ATRIAS_vnmc/control/Virtual Model Control/discrete delay ==
  t : Inport
  Demux : Demux
  Mux : Mux
  Unit Delay{,1..3} (4 alike) : UnitDelay  SampleTime=-1
  t-1 : Outport
  wires:
  Demux/1 -> Unit Delay/1
  t/1 -> Demux/1
  Mux/1 -> t-1/1
  Demux/2 -> Unit Delay1/1
  Unit Delay1/1 -> Mux/2
  Demux/3 -> Unit Delay2/1
  Unit Delay2/1 -> Mux/3
  Demux/4 -> Unit Delay3/1
  Unit Delay3/1 -> Mux/4
  Unit Delay/1 -> Mux/1

== system ATRIAS_vnmc/control/Virtual Model Control/discrete delay1 ==
  t : Inport
  Demux : Demux  Outputs=2
  Mux : Mux  Inputs=2
  Unit Delay : UnitDelay  SampleTime=-1
  Unit Delay1 : UnitDelay  SampleTime=-1
  t-1 : Outport
  wires:
  Unit Delay/1 -> Mux/1
  Unit Delay1/1 -> Mux/2
  Demux/2 -> Unit Delay1/1
  Mux/1 -> t-1/1
  t/1 -> Demux/1
  Demux/1 -> Unit Delay/1

== system ATRIAS_vnmc/control/Virtual Model Control/discrete delay2 ==
  t : Inport
  Demux : Demux  Outputs=2
  Mux : Mux  Inputs=2
  Unit Delay : UnitDelay  SampleTime=-1
  Unit Delay1 : UnitDelay  SampleTime=-1
  t-1 : Outport
  wires:
  Unit Delay/1 -> Mux/1
  Unit Delay1/1 -> Mux/2
  Demux/2 -> Unit Delay1/1
  Mux/1 -> t-1/1
  t/1 -> Demux/1
  Demux/1 -> Unit Delay/1

== system ATRIAS_vnmc/control/Virtual Neuromuscular Control/Higher Control Layer ==
  note: Target Foot Placement
  note: Target Swing Leg Length
      | (constant)
  note: Stance to Swing Leg Decision
  note: Target Trunk Angle
      | (constant)
  note: Higher Control Layer
      | (Supra Spinal Control)
  Double Support : Subsystem
  Mux{1..4} (4 alike) : Mux  Inputs=2
  Sum{1..4} (4 alike) : Sum  Inputs=-+|
  left alpha_tgt (sagittal) : Fcn  Expr=u(1) + u(2)*u(4) + u(3)*u(5)
  right alpha_tgt (sagittal) : Fcn  Expr=u(1) + u(2)*u(4) + u(3)*u(5)
  tag scope: Lalpha_tgt=global, LonR=global, Ralpha_tgt=global, RonL=global, double_support=global, flight=global, leg_clr=global, theta_tgt=global
  wires:
  left alpha_tgt (sagittal)/1 -> [Lalpha_tgt]
  right alpha_tgt (sagittal)/1 -> [Ralpha_tgt]
  [LLCtrlPar] -> [leg_clr]
  Double Support/3(LonR) -> [LonR]
  [LStance] -> Double Support/1(LStance)
  [RStance] -> Double Support/2(RStance)
  Double Support/1(RonL) -> [RonL]
  Double Support/2(Flight) -> [flight]
  Sum1/1 -> Double Support/3(Lalpha_tgt)
  [Lphi23] -> Double Support/4(Lphi34)
  [Rphi23] -> Double Support/7(Rphi34)
  [Lphi12] -> Double Support/5(Lphi23)
  [Rphi12] -> Double Support/8(Rphi23)
  [Lalpha_tgt] -> Sum1/2
  [theta] -> Sum1/1, Sum2/1
  [Ralpha_tgt] -> Sum2/2
  [theta0] -> [theta_tgt]
  Mux1/1 -> left alpha_tgt (sagittal)/1
  [FPCtrlPar] -> Mux4/1, Mux1/1
  Mux2/1 -> Mux1/2
  Mux4/1 -> right alpha_tgt (sagittal)/1
  Mux3/1 -> Mux4/2
  [xRShank1] -> Sum3/1
  [xTorso] -> Sum3/2, Sum4/2
  Sum3/1 -> Mux2/1
  [xLShank1] -> Sum4/1
  Sum4/1 -> Mux3/1
  [dxTorso] -> Mux3/2, Mux2/2
  Double Support/4(DS) -> [double_support]
  Sum2/1 -> Double Support/6(Ralpha_tgt)
